simulink model "HeightModel"  (R2013a)
settings: Solver=ode45  StartTime=0.0  StopTime=30  RelTol=1e-3
values from neighbouring files (symbols this model uses):
  F_yIntercept = -10.4432883127    [Parameters.mat]
  g = 9.81    [Parameters.mat]
  Kf = 9.48907430341    [Parameters.mat]
  Kp_Height = 5.79246370086    [Height_Controller.mat]
  Kw = 501.513336009    [Parameters.mat]
  Mass = 2.26    [MainScriptRoll.m]    (also in Parameters.mat)
  Motor_TimeConstant = 0.07    [Parameters.mat]
  omega_0 = 520    [Yaw_PID.m]
  Speed_yIntercept = -347.939581678    [Parameters.mat]
  T_I = (1/(2*v))*((imag(DCL_Pole_1)/2)-(real(DCL_Pole_1)*v))    [Pitch_Roll_Controller_PID.m]    (also in Yaw_PID.m)
libraries: simulink x3
settings Model: Creator=Ross  LastModifiedBy=Ross

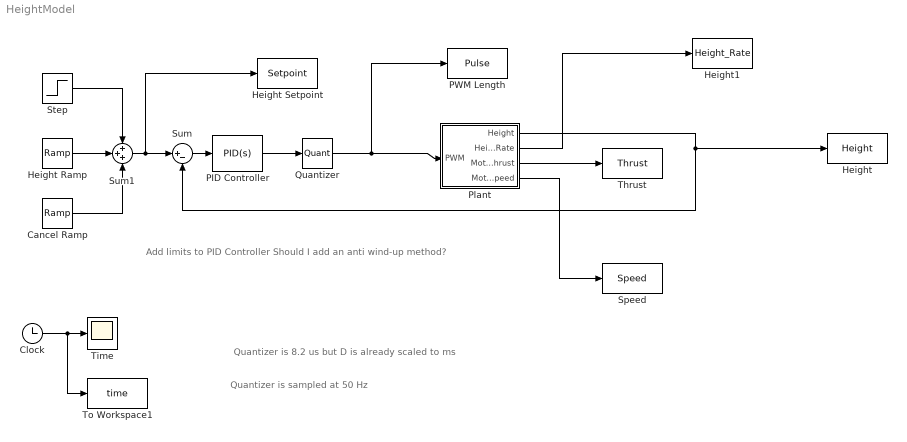
== system HeightModel ==
  note: Quantizer is sampled at 50 Hz
  note: Quantizer is 8.2 us but D
      | is already scaled to ms
  note: Add limits to
      | PID Controller
      | Should I add an anti wind-up method?
  Cancel Ramp : simulink/Sources/Ramp  slope=-1  start=2  X0=0
  Clock : Clock
  Height : ToWorkspace  VariableName=Height  SampleTime=-1  SaveFormat=Timeseries
  Height Ramp : simulink/Sources/Ramp  slope=1  start=1  X0=0
  Height Setpoint : ToWorkspace  VariableName=Setpoint  SampleTime=-1  SaveFormat=Timeseries
  Height1 : ToWorkspace  VariableName=Height_Rate  SampleTime=-1  SaveFormat=Timeseries
  PID Controller : simulink/Continuous/PID Controller  Controller=PID  TimeDomain=Continuous-time  SampleTime=1  IntegratorMethod=Forward Euler  FilterMethod=Forward Euler  Form=Ideal  P=Kp_Height  I=1/T_I  D=T_I/4  N=100  InitialConditionSource=internal  InitialConditionForIntegrator=0  InitialConditionForFilter=0  ExternalReset=none  LimitOutput=on  UpperSaturationLimit=2  LowerSaturationLimit=0  LinearizeAsGain=on  AntiWindupMode=clamping  Kb=1  TrackingMode=off  Kt=1  PParamMin=[]  PParamMax=[]  IParamMin=[]  IParamMax=[]  DParamMin=[]  DParamMax=[]  NParamMin=[]  NParamMax=[]  KbParamMin=[]  KbParamMax=[]  KtParamMin=[]  KtParamMax=[]  POutMin=[]  POutMax=[]  IOutMin=[]  IOutMax=[]  DOutMin=[]  DOutMax=[]  NOutMin=[]  NOutMax=[]  KbOutMin=[]  KbOutMax=[]  KtOutMin=[]  KtOutMax=[]  IntegratorOutMin=[]  IntegratorOutMax=[]  FilterOutMin=[]  FilterOutMax=[]  SumOutMin=[]  SumOutMax=[]  SumI1OutMin=[]  SumI1OutMax=[]  SumI2OutMin=[]  SumI2OutMax=[]  SumI3OutMin=[]  SumI3OutMax=[]  SumDOutMin=[]  SumDOutMax=[]  SaturationOutMin=[]  SaturationOutMax=[]  IntegratorContinuousStateAttributes=''  IntegratorStateMustResolveToSignalObject=off  IntegratorRTWStateStorageClass=Auto  FilterContinuousStateAttributes=''  FilterStateMustResolveToSignalObject=off  FilterRTWStateStorageClass=Auto
  PWM Length : ToWorkspace  VariableName=Pulse  SampleTime=-1  SaveFormat=Timeseries
  Plant : Subsystem
  Quantizer : Quantizer  QuantizationInterval=8.2e-3  SampleTime=0.02
  Speed : ToWorkspace  VariableName=Speed  SampleTime=-1  SaveFormat=Timeseries
  Step : Step  Time=20  SampleTime=0
  Sum : Sum  Inputs=|+-
  Sum1 : Sum  Inputs=+++
  Thrust : ToWorkspace  VariableName=Thrust  SampleTime=-1  SaveFormat=Timeseries
  Time : Scope
  To Workspace1 : ToWorkspace  VariableName=time  SampleTime=-1  SaveFormat=Timeseries
  wires:
  Clock/1 -> To Workspace1/1, Time/1
  Plant/1(Height) -> Sum/2, Height/1
  Sum/1 -> PID Controller/1
  Plant/3(Motor Thrust) -> Thrust/1
  PID Controller/1 -> Quantizer/1
  Sum1/1 -> Height Setpoint/1, Sum/1
  Step/1 -> Sum1/1
  Height Ramp/1 -> Sum1/2
  Cancel Ramp/1 -> Sum1/3
  Quantizer/1 -> PWM Length/1, Plant/1(PWM)
  Plant/4(Motor Speed) -> Speed/1
  Plant/2(HeightRate) -> Height1/1

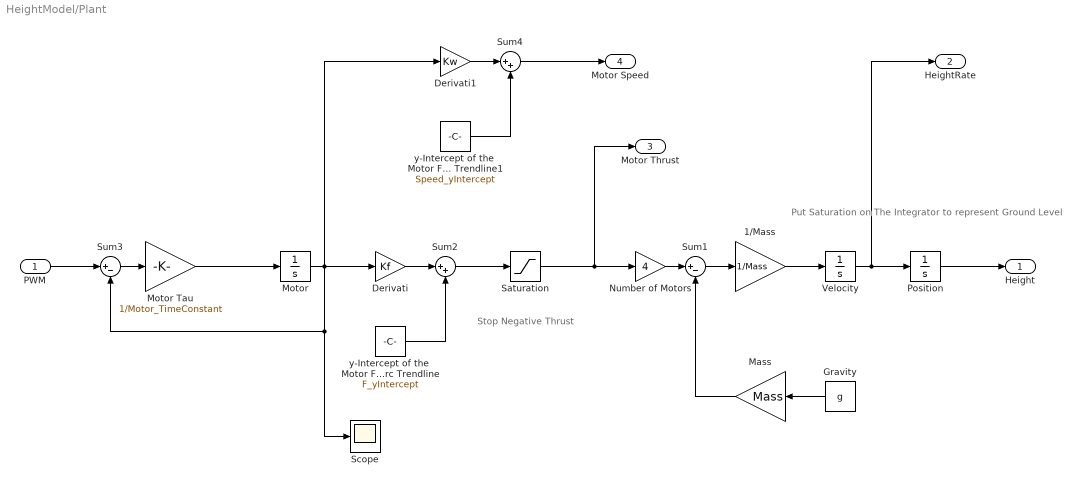
== system HeightModel/Plant ==
  note: Stop Negative
      | Thrust
  note: Put Saturation on
      | The Integrator to represent
      | Ground Level
  PWM : Inport
  1/Mass : Gain  Gain=1/Mass
  Derivati : Gain  Gain=Kf
  Derivati1 : Gain  Gain=Kw
  Gravity : Constant  Value=g
  Mass : Gain  Gain=Mass
  Motor : Integrator  InitialCondition=omega_0
  Motor Tau : Gain  Gain=1/Motor_TimeConstant
  Number of Motors : Gain  Gain=4
  Position : Integrator  LimitOutput=on  LowerSaturationLimit=0
  Saturation : Saturate  UpperLimit=inf  LowerLimit=0
  Scope : Scope
  Sum1 : Sum  Inputs=|+-
  Sum2 : Sum  Inputs=|++
  Sum3 : Sum  Inputs=|+-
  Sum4 : Sum  Inputs=|++
  Velocity : Integrator
  y-Intercept of the  Motor Forc Trendline : Constant  Value=F_yIntercept
  y-Intercept of the  Motor Forc Trendline1 : Constant  Value=Speed_yIntercept
  Height : Outport
  HeightRate : Outport  Port=2
  Motor Thrust : Outport  Port=3
  Motor Speed : Outport  Port=4
  wires:
  Motor Tau/1 -> Motor/1
  Number of Motors/1 -> Sum1/1
  Position/1 -> Height/1
  PWM/1 -> Sum3/1
  Velocity/1 -> HeightRate/1, Position/1
  Sum3/1 -> Motor Tau/1
  1/Mass/1 -> Velocity/1
  Gravity/1 -> Mass/1
  Mass/1 -> Sum1/2
  Sum1/1 -> 1/Mass/1
  Sum2/1 -> Saturation/1
  y-Intercept of the  Motor Forc Trendline/1 -> Sum2/2
  Derivati/1 -> Sum2/1
  Saturation/1 -> Motor Thrust/1, Number of Motors/1
  Motor/1 -> Derivati1/1, Scope/1, Sum3/2, Derivati/1
  Sum4/1 -> Motor Speed/1
  y-Intercept of the  Motor Forc Trendline1/1 -> Sum4/2
  Derivati1/1 -> Sum4/1
